simulink model "TST_DrvDem_SelectParameter"  (R2016b)
settings: Solver=FixedStepDiscrete  StartTime=0.0  StopTime=simTime  FixedStep=sampleTime  RelTol=1e-3
values from neighbouring files (symbols this model uses):
  testCase = 1    [initTST_DrvDem_SelectParameter_001.m]    (also in initTST_DrvDem_SelectParameter_002.m = 2; initTST_DrvDem_SelectParameter_003.m = 3)
libraries: simulink x82, UnitTest_Lib x78
(part 1 of 3)
settings Model: Creator=zhengjinyan  LastModifiedBy=zhengjinyan
settings DebuggingCC: SignalRangeChecking=error

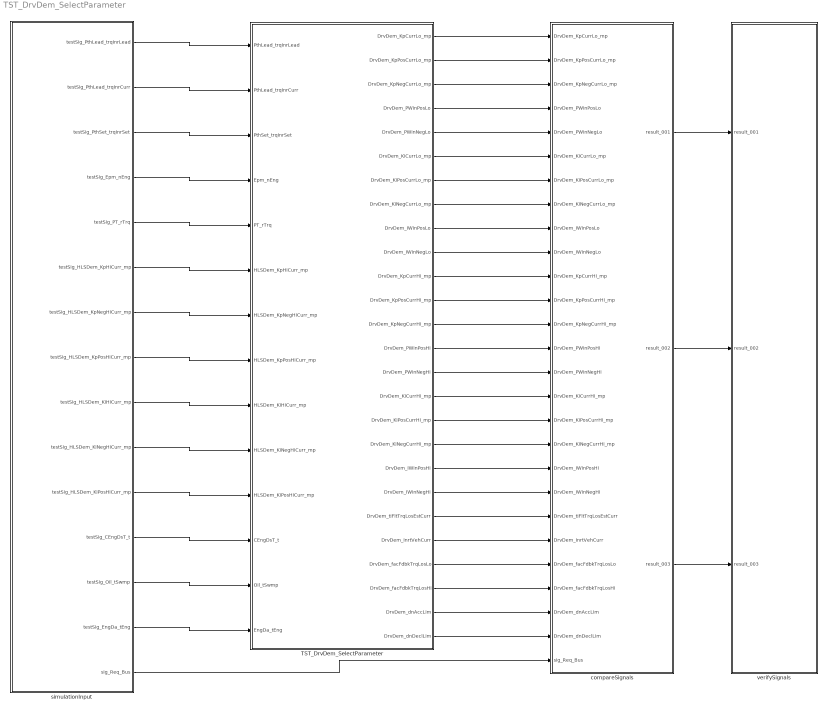
== system TST_DrvDem_SelectParameter ==
  TST_DrvDem_SelectParameter : Subsystem
  compareSignals : Subsystem
  simulationInput : Subsystem
  verifySignals : Subsystem
  wires:
  simulationInput/1(testSig_PthLead_trqInrLead) -> TST_DrvDem_SelectParameter/1(PthLead_trqInrLead)
  simulationInput/2(testSig_PthLead_trqInrCurr) -> TST_DrvDem_SelectParameter/2(PthLead_trqInrCurr)
  simulationInput/3(testSig_PthSet_trqInrSet) -> TST_DrvDem_SelectParameter/3(PthSet_trqInrSet)
  simulationInput/4(testSig_Epm_nEng) -> TST_DrvDem_SelectParameter/4(Epm_nEng)
  simulationInput/5(testSig_PT_rTrq) -> TST_DrvDem_SelectParameter/5(PT_rTrq)
  simulationInput/6(testSig_HLSDem_KpHiCurr_mp) -> TST_DrvDem_SelectParameter/6(HLSDem_KpHiCurr_mp)
  simulationInput/7(testSig_HLSDem_KpNegHiCurr_mp) -> TST_DrvDem_SelectParameter/7(HLSDem_KpNegHiCurr_mp)
  simulationInput/8(testSig_HLSDem_KpPosHiCurr_mp) -> TST_DrvDem_SelectParameter/8(HLSDem_KpPosHiCurr_mp)
  simulationInput/9(testSig_HLSDem_KiHiCurr_mp) -> TST_DrvDem_SelectParameter/9(HLSDem_KiHiCurr_mp)
  simulationInput/10(testSig_HLSDem_KiNegHiCurr_mp) -> TST_DrvDem_SelectParameter/10(HLSDem_KiNegHiCurr_mp)
  simulationInput/11(testSig_HLSDem_KiPosHiCurr_mp) -> TST_DrvDem_SelectParameter/11(HLSDem_KiPosHiCurr_mp)
  simulationInput/12(testSig_CEngDsT_t) -> TST_DrvDem_SelectParameter/12(CEngDsT_t)
  simulationInput/13(testSig_Oil_tSwmp) -> TST_DrvDem_SelectParameter/13(Oil_tSwmp)
  simulationInput/14(testSig_EngDa_tEng) -> TST_DrvDem_SelectParameter/14(EngDa_tEng)
  TST_DrvDem_SelectParameter/1(DrvDem_KpCurrLo_mp) -> compareSignals/1(DrvDem_KpCurrLo_mp)
  TST_DrvDem_SelectParameter/2(DrvDem_KpPosCurrLo_mp) -> compareSignals/2(DrvDem_KpPosCurrLo_mp)
  TST_DrvDem_SelectParameter/3(DrvDem_KpNegCurrLo_mp) -> compareSignals/3(DrvDem_KpNegCurrLo_mp)
  TST_DrvDem_SelectParameter/4(DrvDem_PWinPosLo) -> compareSignals/4(DrvDem_PWinPosLo)
  TST_DrvDem_SelectParameter/5(DrvDem_PWinNegLo) -> compareSignals/5(DrvDem_PWinNegLo)
  TST_DrvDem_SelectParameter/6(DrvDem_KiCurrLo_mp) -> compareSignals/6(DrvDem_KiCurrLo_mp)
  TST_DrvDem_SelectParameter/7(DrvDem_KiPosCurrLo_mp) -> compareSignals/7(DrvDem_KiPosCurrLo_mp)
  TST_DrvDem_SelectParameter/8(DrvDem_KiNegCurrLo_mp) -> compareSignals/8(DrvDem_KiNegCurrLo_mp)
  TST_DrvDem_SelectParameter/9(DrvDem_IWinPosLo) -> compareSignals/9(DrvDem_IWinPosLo)
  TST_DrvDem_SelectParameter/10(DrvDem_IWinNegLo) -> compareSignals/10(DrvDem_IWinNegLo)
  TST_DrvDem_SelectParameter/11(DrvDem_KpCurrHi_mp) -> compareSignals/11(DrvDem_KpCurrHi_mp)
  TST_DrvDem_SelectParameter/12(DrvDem_KpPosCurrHi_mp) -> compareSignals/12(DrvDem_KpPosCurrHi_mp)
  TST_DrvDem_SelectParameter/13(DrvDem_KpNegCurrHi_mp) -> compareSignals/13(DrvDem_KpNegCurrHi_mp)
  TST_DrvDem_SelectParameter/14(DrvDem_PWinPosHi) -> compareSignals/14(DrvDem_PWinPosHi)
  TST_DrvDem_SelectParameter/15(DrvDem_PWinNegHi) -> compareSignals/15(DrvDem_PWinNegHi)
  TST_DrvDem_SelectParameter/16(DrvDem_KiCurrHi_mp) -> compareSignals/16(DrvDem_KiCurrHi_mp)
  TST_DrvDem_SelectParameter/17(DrvDem_KiPosCurrHi_mp) -> compareSignals/17(DrvDem_KiPosCurrHi_mp)
  TST_DrvDem_SelectParameter/18(DrvDem_KiNegCurrHi_mp) -> compareSignals/18(DrvDem_KiNegCurrHi_mp)
  TST_DrvDem_SelectParameter/19(DrvDem_IWinPosHi) -> compareSignals/19(DrvDem_IWinPosHi)
  TST_DrvDem_SelectParameter/20(DrvDem_IWinNegHi) -> compareSignals/20(DrvDem_IWinNegHi)
  TST_DrvDem_SelectParameter/21(DrvDem_tiFltTrqLosEstCurr) -> compareSignals/21(DrvDem_tiFltTrqLosEstCurr)
  TST_DrvDem_SelectParameter/22(DrvDem_InrtVehCurr) -> compareSignals/22(DrvDem_InrtVehCurr)
  TST_DrvDem_SelectParameter/23(DrvDem_facFdbkTrqLosLo) -> compareSignals/23(DrvDem_facFdbkTrqLosLo)
  TST_DrvDem_SelectParameter/24(DrvDem_facFdbkTrqLosHi) -> compareSignals/24(DrvDem_facFdbkTrqLosHi)
  TST_DrvDem_SelectParameter/25(DrvDem_dnAccLim) -> compareSignals/25(DrvDem_dnAccLim)
  TST_DrvDem_SelectParameter/26(DrvDem_dnDeclLim) -> compareSignals/26(DrvDem_dnDeclLim)
  simulationInput/15(sig_Req_Bus) -> compareSignals/27(sig_Req_Bus)
  compareSignals/1(result_001) -> verifySignals/1(result_001)
  compareSignals/2(result_002) -> verifySignals/2(result_002)
  compareSignals/3(result_003) -> verifySignals/3(result_003)

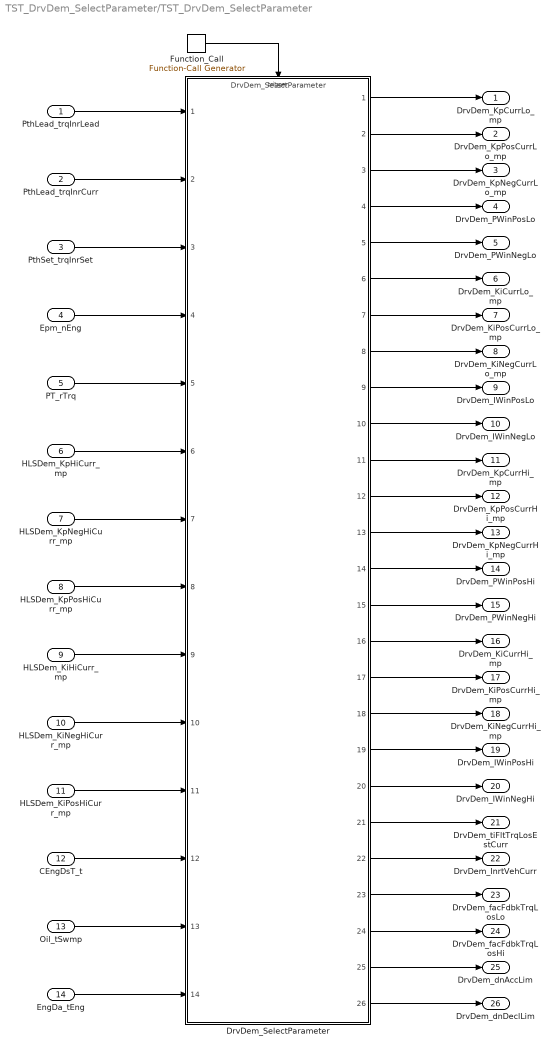
== system TST_DrvDem_SelectParameter/TST_DrvDem_SelectParameter ==
  PthLead_trqInrLead : Inport
  PthLead_trqInrCurr : Inport  Port=2
  PthSet_trqInrSet : Inport  Port=3
  Epm_nEng : Inport  Port=4
  PT_rTrq : Inport  Port=5
  HLSDem_KpHiCurr_mp : Inport  Port=6
  HLSDem_KpNegHiCurr_mp : Inport  Port=7
  HLSDem_KpPosHiCurr_mp : Inport  Port=8
  HLSDem_KiHiCurr_mp : Inport  Port=9
  HLSDem_KiNegHiCurr_mp : Inport  Port=10
  HLSDem_KiPosHiCurr_mp : Inport  Port=11
  CEngDsT_t : Inport  Port=12
  Oil_tSwmp : Inport  Port=13
  EngDa_tEng : Inport  Port=14
  DrvDem_SelectParameter : ModelReference  ModelNameDialog=DrvDem_SelectParameter  SimulationMode=Normal  ModelReferenceVersion=1.41  TriggerPortName=function  TriggerPortTriggerType=function-call  TriggerPortStatesWhenEnabling=held
  Function_Call : simulink/Ports & Subsystems/Function-Call Generator  sample_time=sampleTime  numberOfIterations=1
  DrvDem_KpCurrLo_mp : Outport
  DrvDem_KpPosCurrLo_mp : Outport  Port=2
  DrvDem_KpNegCurrLo_mp : Outport  Port=3
  DrvDem_PWinPosLo : Outport  Port=4
  DrvDem_PWinNegLo : Outport  Port=5
  DrvDem_KiCurrLo_mp : Outport  Port=6
  DrvDem_KiPosCurrLo_mp : Outport  Port=7
  DrvDem_KiNegCurrLo_mp : Outport  Port=8
  DrvDem_IWinPosLo : Outport  Port=9
  DrvDem_IWinNegLo : Outport  Port=10
  DrvDem_KpCurrHi_mp : Outport  Port=11
  DrvDem_KpPosCurrHi_mp : Outport  Port=12
  DrvDem_KpNegCurrHi_mp : Outport  Port=13
  DrvDem_PWinPosHi : Outport  Port=14
  DrvDem_PWinNegHi : Outport  Port=15
  DrvDem_KiCurrHi_mp : Outport  Port=16
  DrvDem_KiPosCurrHi_mp : Outport  Port=17
  DrvDem_KiNegCurrHi_mp : Outport  Port=18
  DrvDem_IWinPosHi : Outport  Port=19
  DrvDem_IWinNegHi : Outport  Port=20
  DrvDem_tiFltTrqLosEstCurr : Outport  Port=21
  DrvDem_InrtVehCurr : Outport  Port=22
  DrvDem_facFdbkTrqLosLo : Outport  Port=23
  DrvDem_facFdbkTrqLosHi : Outport  Port=24
  DrvDem_dnAccLim : Outport  Port=25
  DrvDem_dnDeclLim : Outport  Port=26
  wires:
  Function_Call/1 -> DrvDem_SelectParameter/Trigger
  PthLead_trqInrLead/1 -> DrvDem_SelectParameter/1
  PthLead_trqInrCurr/1 -> DrvDem_SelectParameter/2
  PthSet_trqInrSet/1 -> DrvDem_SelectParameter/3
  Epm_nEng/1 -> DrvDem_SelectParameter/4
  PT_rTrq/1 -> DrvDem_SelectParameter/5
  HLSDem_KpHiCurr_mp/1 -> DrvDem_SelectParameter/6
  HLSDem_KpNegHiCurr_mp/1 -> DrvDem_SelectParameter/7
  HLSDem_KpPosHiCurr_mp/1 -> DrvDem_SelectParameter/8
  HLSDem_KiHiCurr_mp/1 -> DrvDem_SelectParameter/9
  HLSDem_KiNegHiCurr_mp/1 -> DrvDem_SelectParameter/10
  HLSDem_KiPosHiCurr_mp/1 -> DrvDem_SelectParameter/11
  CEngDsT_t/1 -> DrvDem_SelectParameter/12
  Oil_tSwmp/1 -> DrvDem_SelectParameter/13
  EngDa_tEng/1 -> DrvDem_SelectParameter/14
  DrvDem_SelectParameter/1 -> DrvDem_KpCurrLo_mp/1
  DrvDem_SelectParameter/2 -> DrvDem_KpPosCurrLo_mp/1
  DrvDem_SelectParameter/3 -> DrvDem_KpNegCurrLo_mp/1
  DrvDem_SelectParameter/4 -> DrvDem_PWinPosLo/1
  DrvDem_SelectParameter/5 -> DrvDem_PWinNegLo/1
  DrvDem_SelectParameter/6 -> DrvDem_KiCurrLo_mp/1
  DrvDem_SelectParameter/7 -> DrvDem_KiPosCurrLo_mp/1
  DrvDem_SelectParameter/8 -> DrvDem_KiNegCurrLo_mp/1
  DrvDem_SelectParameter/9 -> DrvDem_IWinPosLo/1
  DrvDem_SelectParameter/10 -> DrvDem_IWinNegLo/1
  DrvDem_SelectParameter/11 -> DrvDem_KpCurrHi_mp/1
  DrvDem_SelectParameter/12 -> DrvDem_KpPosCurrHi_mp/1
  DrvDem_SelectParameter/13 -> DrvDem_KpNegCurrHi_mp/1
  DrvDem_SelectParameter/14 -> DrvDem_PWinPosHi/1
  DrvDem_SelectParameter/15 -> DrvDem_PWinNegHi/1
  DrvDem_SelectParameter/16 -> DrvDem_KiCurrHi_mp/1
  DrvDem_SelectParameter/17 -> DrvDem_KiPosCurrHi_mp/1
  DrvDem_SelectParameter/18 -> DrvDem_KiNegCurrHi_mp/1
  DrvDem_SelectParameter/19 -> DrvDem_IWinPosHi/1
  DrvDem_SelectParameter/20 -> DrvDem_IWinNegHi/1
  DrvDem_SelectParameter/21 -> DrvDem_tiFltTrqLosEstCurr/1
  DrvDem_SelectParameter/22 -> DrvDem_InrtVehCurr/1
  DrvDem_SelectParameter/23 -> DrvDem_facFdbkTrqLosLo/1
  DrvDem_SelectParameter/24 -> DrvDem_facFdbkTrqLosHi/1
  DrvDem_SelectParameter/25 -> DrvDem_dnAccLim/1
  DrvDem_SelectParameter/26 -> DrvDem_dnDeclLim/1

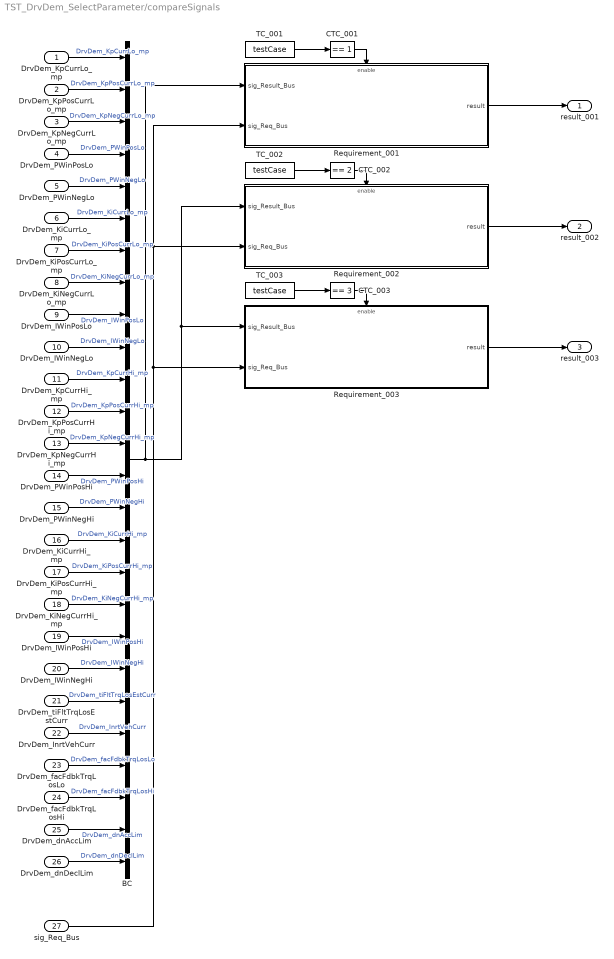
== system TST_DrvDem_SelectParameter/compareSignals ==
  DrvDem_KpCurrLo_mp : Inport
  DrvDem_KpPosCurrLo_mp : Inport  Port=2
  DrvDem_KpNegCurrLo_mp : Inport  Port=3
  DrvDem_PWinPosLo : Inport  Port=4
  DrvDem_PWinNegLo : Inport  Port=5
  DrvDem_KiCurrLo_mp : Inport  Port=6
  DrvDem_KiPosCurrLo_mp : Inport  Port=7
  DrvDem_KiNegCurrLo_mp : Inport  Port=8
  DrvDem_IWinPosLo : Inport  Port=9
  DrvDem_IWinNegLo : Inport  Port=10
  DrvDem_KpCurrHi_mp : Inport  Port=11
  DrvDem_KpPosCurrHi_mp : Inport  Port=12
  DrvDem_KpNegCurrHi_mp : Inport  Port=13
  DrvDem_PWinPosHi : Inport  Port=14
  DrvDem_PWinNegHi : Inport  Port=15
  DrvDem_KiCurrHi_mp : Inport  Port=16
  DrvDem_KiPosCurrHi_mp : Inport  Port=17
  DrvDem_KiNegCurrHi_mp : Inport  Port=18
  DrvDem_IWinPosHi : Inport  Port=19
  DrvDem_IWinNegHi : Inport  Port=20
  DrvDem_tiFltTrqLosEstCurr : Inport  Port=21
  DrvDem_InrtVehCurr : Inport  Port=22
  DrvDem_facFdbkTrqLosLo : Inport  Port=23
  DrvDem_facFdbkTrqLosHi : Inport  Port=24
  DrvDem_dnAccLim : Inport  Port=25
  DrvDem_dnDeclLim : Inport  Port=26
  sig_Req_Bus : Inport  Port=27
  BC : BusCreator  Inputs=26
  CTC_001 : simulink/Logic and Bit Operations/Compare To Constant  relop===  const=1  OutDataTypeStr=boolean
  CTC_002 : simulink/Logic and Bit Operations/Compare To Constant  relop===  const=2  OutDataTypeStr=boolean
  CTC_003 : simulink/Logic and Bit Operations/Compare To Constant  relop===  const=3  OutDataTypeStr=boolean
  Requirement_001 : Subsystem
  Requirement_002 : Subsystem
  Requirement_003 : Subsystem
  TC_001 : Constant  Value=testCase
  TC_002 : Constant  Value=testCase
  TC_003 : Constant  Value=testCase
  result_001 : Outport
  result_002 : Outport  Port=2
  result_003 : Outport  Port=3
  wires:
  DrvDem_KpCurrLo_mp/1 -> BC/1  "DrvDem_KpCurrLo_mp"
  DrvDem_KpPosCurrLo_mp/1 -> BC/2  "DrvDem_KpPosCurrLo_mp"
  DrvDem_KpNegCurrLo_mp/1 -> BC/3  "DrvDem_KpNegCurrLo_mp"
  DrvDem_PWinPosLo/1 -> BC/4  "DrvDem_PWinPosLo"
  DrvDem_PWinNegLo/1 -> BC/5  "DrvDem_PWinNegLo"
  DrvDem_KiCurrLo_mp/1 -> BC/6  "DrvDem_KiCurrLo_mp"
  DrvDem_KiPosCurrLo_mp/1 -> BC/7  "DrvDem_KiPosCurrLo_mp"
  DrvDem_KiNegCurrLo_mp/1 -> BC/8  "DrvDem_KiNegCurrLo_mp"
  DrvDem_IWinPosLo/1 -> BC/9  "DrvDem_IWinPosLo"
  DrvDem_IWinNegLo/1 -> BC/10  "DrvDem_IWinNegLo"
  DrvDem_KpCurrHi_mp/1 -> BC/11  "DrvDem_KpCurrHi_mp"
  DrvDem_KpPosCurrHi_mp/1 -> BC/12  "DrvDem_KpPosCurrHi_mp"
  DrvDem_KpNegCurrHi_mp/1 -> BC/13  "DrvDem_KpNegCurrHi_mp"
  DrvDem_PWinPosHi/1 -> BC/14  "DrvDem_PWinPosHi"
  DrvDem_PWinNegHi/1 -> BC/15  "DrvDem_PWinNegHi"
  DrvDem_KiCurrHi_mp/1 -> BC/16  "DrvDem_KiCurrHi_mp"
  DrvDem_KiPosCurrHi_mp/1 -> BC/17  "DrvDem_KiPosCurrHi_mp"
  DrvDem_KiNegCurrHi_mp/1 -> BC/18  "DrvDem_KiNegCurrHi_mp"
  DrvDem_IWinPosHi/1 -> BC/19  "DrvDem_IWinPosHi"
  DrvDem_IWinNegHi/1 -> BC/20  "DrvDem_IWinNegHi"
  DrvDem_tiFltTrqLosEstCurr/1 -> BC/21  "DrvDem_tiFltTrqLosEstCurr"
  DrvDem_InrtVehCurr/1 -> BC/22  "DrvDem_InrtVehCurr"
  DrvDem_facFdbkTrqLosLo/1 -> BC/23  "DrvDem_facFdbkTrqLosLo"
  DrvDem_facFdbkTrqLosHi/1 -> BC/24  "DrvDem_facFdbkTrqLosHi"
  DrvDem_dnAccLim/1 -> BC/25  "DrvDem_dnAccLim"
  DrvDem_dnDeclLim/1 -> BC/26  "DrvDem_dnDeclLim"
  TC_001/1 -> CTC_001/1
  CTC_001/1 -> Requirement_001/Enable
  sig_Req_Bus/1 -> Requirement_001/2(sig_Req_Bus), Requirement_002/2(sig_Req_Bus), Requirement_003/2(sig_Req_Bus)
  BC/1 -> Requirement_002/1(sig_Result_Bus), Requirement_003/1(sig_Result_Bus), Requirement_001/1(sig_Result_Bus)
  Requirement_001/1(result) -> result_001/1
  TC_002/1 -> CTC_002/1
  CTC_002/1 -> Requirement_002/Enable
  Requirement_002/1(result) -> result_002/1
  TC_003/1 -> CTC_003/1
  CTC_003/1 -> Requirement_003/Enable
  Requirement_003/1(result) -> result_003/1

== system TST_DrvDem_SelectParameter/simulationInput ==
  BS : BusSelector  OutputSignals=testSig_PthLead_trqInrLead,testSig_PthLead_trqInrCurr,testSig_PthSet_trqInrSet,testSig_Epm_nEng,testSig_PT_rTrq,testSig_HLSDem_KpHiCurr_mp,testSig_HLSDem_KpNegHiCurr_mp,testSig_HLSDem_KpPosHiCurr_mp,testSig_HLSDem_KiHiCurr_mp,testSig_HLSDem_KiNegHiCurr_mp,testSig_HLSDem_KiPosHiCurr_mp,testSig_CEngDsT_t,testSig_Oil_tSwmp,testSig_EngDa_tEng
  MPSw : MultiPortSwitch  SaturateOnIntegerOverflow=on  InputSameDT=on
  TestCase : Constant  Value=testCase
  testSignals_R001 : Subsystem
  testSignals_R002 : Subsystem
  testSignals_R003 : Subsystem
  testSig_PthLead_trqInrLead : Outport
  testSig_PthLead_trqInrCurr : Outport  Port=2
  testSig_PthSet_trqInrSet : Outport  Port=3
  testSig_Epm_nEng : Outport  Port=4
  testSig_PT_rTrq : Outport  Port=5
  testSig_HLSDem_KpHiCurr_mp : Outport  Port=6
  testSig_HLSDem_KpNegHiCurr_mp : Outport  Port=7
  testSig_HLSDem_KpPosHiCurr_mp : Outport  Port=8
  testSig_HLSDem_KiHiCurr_mp : Outport  Port=9
  testSig_HLSDem_KiNegHiCurr_mp : Outport  Port=10
  testSig_HLSDem_KiPosHiCurr_mp : Outport  Port=11
  testSig_CEngDsT_t : Outport  Port=12
  testSig_Oil_tSwmp : Outport  Port=13
  testSig_EngDa_tEng : Outport  Port=14
  sig_Req_Bus : Outport  Port=15
  wires:
  BS/1 -> testSig_PthLead_trqInrLead/1  "<testSig_PthLead_trqInrLead>"
  BS/2 -> testSig_PthLead_trqInrCurr/1  "<testSig_PthLead_trqInrCurr>"
  BS/3 -> testSig_PthSet_trqInrSet/1  "<testSig_PthSet_trqInrSet>"
  BS/4 -> testSig_Epm_nEng/1  "<testSig_Epm_nEng>"
  BS/5 -> testSig_PT_rTrq/1  "<testSig_PT_rTrq>"
  BS/6 -> testSig_HLSDem_KpHiCurr_mp/1  "<testSig_HLSDem_KpHiCurr_mp>"
  BS/7 -> testSig_HLSDem_KpNegHiCurr_mp/1  "<testSig_HLSDem_KpNegHiCurr_mp>"
  BS/8 -> testSig_HLSDem_KpPosHiCurr_mp/1  "<testSig_HLSDem_KpPosHiCurr_mp>"
  BS/9 -> testSig_HLSDem_KiHiCurr_mp/1  "<testSig_HLSDem_KiHiCurr_mp>"
  BS/10 -> testSig_HLSDem_KiNegHiCurr_mp/1  "<testSig_HLSDem_KiNegHiCurr_mp>"
  BS/11 -> testSig_HLSDem_KiPosHiCurr_mp/1  "<testSig_HLSDem_KiPosHiCurr_mp>"
  BS/12 -> testSig_CEngDsT_t/1  "<testSig_CEngDsT_t>"
  BS/13 -> testSig_Oil_tSwmp/1  "<testSig_Oil_tSwmp>"
  BS/14 -> testSig_EngDa_tEng/1  "<testSig_EngDa_tEng>"
  MPSw/1 -> BS/1, sig_Req_Bus/1
  TestCase/1 -> MPSw/1
  testSignals_R001/1(testSignals) -> MPSw/2
  testSignals_R002/1(testSignals) -> MPSw/3
  testSignals_R003/1(testSignals) -> MPSw/4

== system TST_DrvDem_SelectParameter/verifySignals ==
  result_001 : Inport
  result_002 : Inport  Port=2
  result_003 : Inport  Port=3
  Assertion_001 : Assertion  Enabled=off
  Assertion_002 : Assertion  Enabled=off
  Assertion_003 : Assertion  Enabled=off
  wires:
  result_001/1 -> Assertion_001/1
  result_002/1 -> Assertion_002/1
  result_003/1 -> Assertion_003/1

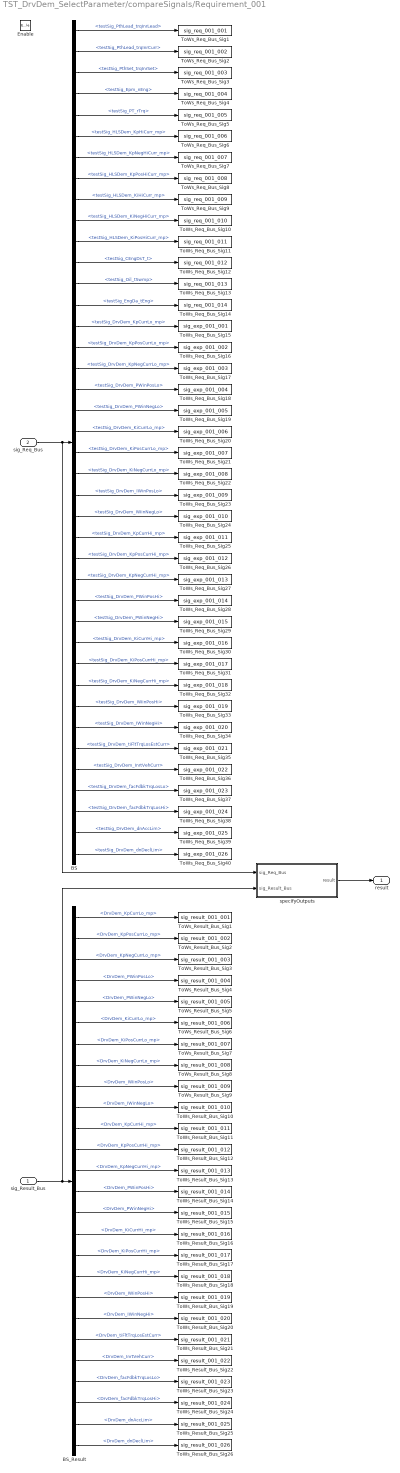
== system TST_DrvDem_SelectParameter/compareSignals/Requirement_001 ==
  sig_Result_Bus : Inport
  sig_Req_Bus : Inport  Port=2
  Enable : EnablePort
  BS : BusSelector  OutputSignals=testSig_PthLead_trqInrLead,testSig_PthLead_trqInrCurr,testSig_PthSet_trqInrSet,testSig_Epm_nEng,testSig_PT_rTrq,testSig_HLSDem_KpHiCurr_mp,testSig_HLSDem_KpNegHiCurr_mp,testSig_HLSDem_KpPosHiCurr_mp,testSig_HLSDem_KiHiCurr_mp,testSig_HLSDem_KiNegHiCurr_mp,testSig_HLSDem_KiPosHiCurr_mp,testSig_CEngDsT_t,testSig_Oil_tSwmp,testSig_EngDa_tEng,testSig_DrvDem_KpCurrLo_mp,testSig_DrvDem_KpPosCurrLo_mp,testSig_DrvDem_KpNegCurrLo_mp,testSig_DrvDem_PWinPosLo,testSig_DrvDem_PWinNegLo,testSig_DrvDem_KiCurrLo_mp,testSig_DrvDem_KiPosCurrLo_mp,testSig_DrvDem_KiNegCurrLo_mp,testSig_DrvDem_IWinPosLo,testSig_DrvDem_IWinNegLo,testSig_DrvDem_KpCurrHi_mp,testSig_DrvDem_KpPosCurrHi_mp,testSig_DrvDem_KpNegCurrHi_mp,testSig_DrvDem_PWinPosHi,testSig_DrvDem_PWinNegHi,testSig_DrvDem_KiCurrHi_mp,testSig_DrvDem_KiPosCurrHi_mp,testSig_DrvDem_KiNegCurrHi_mp,testSig_DrvDem_IWinPosHi,testSig_DrvDem_IWinNegHi,testSig_DrvDem_tiFltTrqLosEstCurr,testSig_DrvDem_InrtVehCurr,testSig_DrvDem_facFdbkTrqLosLo,testSig_DrvDem_facFdbkTrqLosHi,testSig_DrvDem_dnAccLim,testSig_DrvDem_dnDeclLim
  BS_Result : BusSelector  OutputSignals=DrvDem_KpCurrLo_mp,DrvDem_KpPosCurrLo_mp,DrvDem_KpNegCurrLo_mp,DrvDem_PWinPosLo,DrvDem_PWinNegLo,DrvDem_KiCurrLo_mp,DrvDem_KiPosCurrLo_mp,DrvDem_KiNegCurrLo_mp,DrvDem_IWinPosLo,DrvDem_IWinNegLo,DrvDem_KpCurrHi_mp,DrvDem_KpPosCurrHi_mp,DrvDem_KpNegCurrHi_mp,DrvDem_PWinPosHi,DrvDem_PWinNegHi,DrvDem_KiCurrHi_mp,DrvDem_KiPosCurrHi_mp,DrvDem_KiNegCurrHi_mp,DrvDem_IWinPosHi,DrvDem_IWinNegHi,DrvDem_tiFltTrqLosEstCurr,DrvDem_InrtVehCurr,DrvDem_facFdbkTrqLosLo,DrvDem_facFdbkTrqLosHi,DrvDem_dnAccLim,DrvDem_dnDeclLim
  ToWs_Req_Bus_Sig1 : ToWorkspace  VariableName=sig_req_001_001  SaveFormat=Structure With Time
  ToWs_Req_Bus_Sig10 : ToWorkspace  VariableName=sig_req_001_010  SaveFormat=Structure With Time
  ToWs_Req_Bus_Sig11 : ToWorkspace  VariableName=sig_req_001_011  SaveFormat=Structure With Time
  ToWs_Req_Bus_Sig12 : ToWorkspace  VariableName=sig_req_001_012  SaveFormat=Structure With Time
  ToWs_Req_Bus_Sig13 : ToWorkspace  VariableName=sig_req_001_013  SaveFormat=Structure With Time
  ToWs_Req_Bus_Sig14 : ToWorkspace  VariableName=sig_req_001_014  SaveFormat=Structure With Time
  ToWs_Req_Bus_Sig15 : ToWorkspace  VariableName=sig_exp_001_001  SaveFormat=Structure With Time
  ToWs_Req_Bus_Sig16 : ToWorkspace  VariableName=sig_exp_001_002  SaveFormat=Structure With Time
  ToWs_Req_Bus_Sig17 : ToWorkspace  VariableName=sig_exp_001_003  SaveFormat=Structure With Time
  ToWs_Req_Bus_Sig18 : ToWorkspace  VariableName=sig_exp_001_004  SaveFormat=Structure With Time
  ToWs_Req_Bus_Sig19 : ToWorkspace  VariableName=sig_exp_001_005  SaveFormat=Structure With Time
  ToWs_Req_Bus_Sig2 : ToWorkspace  VariableName=sig_req_001_002  SaveFormat=Structure With Time
  ToWs_Req_Bus_Sig20 : ToWorkspace  VariableName=sig_exp_001_006  SaveFormat=Structure With Time
  ToWs_Req_Bus_Sig21 : ToWorkspace  VariableName=sig_exp_001_007  SaveFormat=Structure With Time
  ToWs_Req_Bus_Sig22 : ToWorkspace  VariableName=sig_exp_001_008  SaveFormat=Structure With Time
  ToWs_Req_Bus_Sig23 : ToWorkspace  VariableName=sig_exp_001_009  SaveFormat=Structure With Time
  ToWs_Req_Bus_Sig24 : ToWorkspace  VariableName=sig_exp_001_010  SaveFormat=Structure With Time
  ToWs_Req_Bus_Sig25 : ToWorkspace  VariableName=sig_exp_001_011  SaveFormat=Structure With Time
  ToWs_Req_Bus_Sig26 : ToWorkspace  VariableName=sig_exp_001_012  SaveFormat=Structure With Time
  ToWs_Req_Bus_Sig27 : ToWorkspace  VariableName=sig_exp_001_013  SaveFormat=Structure With Time
  ToWs_Req_Bus_Sig28 : ToWorkspace  VariableName=sig_exp_001_014  SaveFormat=Structure With Time
  ToWs_Req_Bus_Sig29 : ToWorkspace  VariableName=sig_exp_001_015  SaveFormat=Structure With Time
  ToWs_Req_Bus_Sig3 : ToWorkspace  VariableName=sig_req_001_003  SaveFormat=Structure With Time
  ToWs_Req_Bus_Sig30 : ToWorkspace  VariableName=sig_exp_001_016  SaveFormat=Structure With Time
  ToWs_Req_Bus_Sig31 : ToWorkspace  VariableName=sig_exp_001_017  SaveFormat=Structure With Time
  ToWs_Req_Bus_Sig32 : ToWorkspace  VariableName=sig_exp_001_018  SaveFormat=Structure With Time
  ToWs_Req_Bus_Sig33 : ToWorkspace  VariableName=sig_exp_001_019  SaveFormat=Structure With Time
  ToWs_Req_Bus_Sig34 : ToWorkspace  VariableName=sig_exp_001_020  SaveFormat=Structure With Time
  ToWs_Req_Bus_Sig35 : ToWorkspace  VariableName=sig_exp_001_021  SaveFormat=Structure With Time
  ToWs_Req_Bus_Sig36 : ToWorkspace  VariableName=sig_exp_001_022  SaveFormat=Structure With Time
  ToWs_Req_Bus_Sig37 : ToWorkspace  VariableName=sig_exp_001_023  SaveFormat=Structure With Time
  ToWs_Req_Bus_Sig38 : ToWorkspace  VariableName=sig_exp_001_024  SaveFormat=Structure With Time
  ToWs_Req_Bus_Sig39 : ToWorkspace  VariableName=sig_exp_001_025  SaveFormat=Structure With Time
  ToWs_Req_Bus_Sig4 : ToWorkspace  VariableName=sig_req_001_004  SaveFormat=Structure With Time
  ToWs_Req_Bus_Sig40 : ToWorkspace  VariableName=sig_exp_001_026  SaveFormat=Structure With Time
  ToWs_Req_Bus_Sig5 : ToWorkspace  VariableName=sig_req_001_005  SaveFormat=Structure With Time
  ToWs_Req_Bus_Sig6 : ToWorkspace  VariableName=sig_req_001_006  SaveFormat=Structure With Time
  ToWs_Req_Bus_Sig7 : ToWorkspace  VariableName=sig_req_001_007  SaveFormat=Structure With Time
  ToWs_Req_Bus_Sig8 : ToWorkspace  VariableName=sig_req_001_008  SaveFormat=Structure With Time
  ToWs_Req_Bus_Sig9 : ToWorkspace  VariableName=sig_req_001_009  SaveFormat=Structure With Time
  ToWs_Result_Bus_Sig1 : ToWorkspace  VariableName=sig_result_001_001  SaveFormat=Structure With Time
  ToWs_Result_Bus_Sig10 : ToWorkspace  VariableName=sig_result_001_010  SaveFormat=Structure With Time
  ToWs_Result_Bus_Sig11 : ToWorkspace  VariableName=sig_result_001_011  SaveFormat=Structure With Time
  ToWs_Result_Bus_Sig12 : ToWorkspace  VariableName=sig_result_001_012  SaveFormat=Structure With Time
  ToWs_Result_Bus_Sig13 : ToWorkspace  VariableName=sig_result_001_013  SaveFormat=Structure With Time
  ToWs_Result_Bus_Sig14 : ToWorkspace  VariableName=sig_result_001_014  SaveFormat=Structure With Time
  ToWs_Result_Bus_Sig15 : ToWorkspace  VariableName=sig_result_001_015  SaveFormat=Structure With Time
  ToWs_Result_Bus_Sig16 : ToWorkspace  VariableName=sig_result_001_016  SaveFormat=Structure With Time
  ToWs_Result_Bus_Sig17 : ToWorkspace  VariableName=sig_result_001_017  SaveFormat=Structure With Time
  ToWs_Result_Bus_Sig18 : ToWorkspace  VariableName=sig_result_001_018  SaveFormat=Structure With Time
  ToWs_Result_Bus_Sig19 : ToWorkspace  VariableName=sig_result_001_019  SaveFormat=Structure With Time
  ToWs_Result_Bus_Sig2 : ToWorkspace  VariableName=sig_result_001_002  SaveFormat=Structure With Time
  ToWs_Result_Bus_Sig20 : ToWorkspace  VariableName=sig_result_001_020  SaveFormat=Structure With Time
  ToWs_Result_Bus_Sig21 : ToWorkspace  VariableName=sig_result_001_021  SaveFormat=Structure With Time
  ToWs_Result_Bus_Sig22 : ToWorkspace  VariableName=sig_result_001_022  SaveFormat=Structure With Time
  ToWs_Result_Bus_Sig23 : ToWorkspace  VariableName=sig_result_001_023  SaveFormat=Structure With Time
  ToWs_Result_Bus_Sig24 : ToWorkspace  VariableName=sig_result_001_024  SaveFormat=Structure With Time
  ToWs_Result_Bus_Sig25 : ToWorkspace  VariableName=sig_result_001_025  SaveFormat=Structure With Time
  ToWs_Result_Bus_Sig26 : ToWorkspace  VariableName=sig_result_001_026  SaveFormat=Structure With Time
  ToWs_Result_Bus_Sig3 : ToWorkspace  VariableName=sig_result_001_003  SaveFormat=Structure With Time
  ToWs_Result_Bus_Sig4 : ToWorkspace  VariableName=sig_result_001_004  SaveFormat=Structure With Time
  ToWs_Result_Bus_Sig5 : ToWorkspace  VariableName=sig_result_001_005  SaveFormat=Structure With Time
  ToWs_Result_Bus_Sig6 : ToWorkspace  VariableName=sig_result_001_006  SaveFormat=Structure With Time
  ToWs_Result_Bus_Sig7 : ToWorkspace  VariableName=sig_result_001_007  SaveFormat=Structure With Time
  ToWs_Result_Bus_Sig8 : ToWorkspace  VariableName=sig_result_001_008  SaveFormat=Structure With Time
  ToWs_Result_Bus_Sig9 : ToWorkspace  VariableName=sig_result_001_009  SaveFormat=Structure With Time
  specifyOutputs : Subsystem
  result : Outport
  wires:
  sig_Req_Bus/1 -> BS/1, specifyOutputs/1(sig_Req_Bus)
  BS/1 -> ToWs_Req_Bus_Sig1/1  "<testSig_PthLead_trqInrLead>"
  BS/2 -> ToWs_Req_Bus_Sig2/1  "<testSig_PthLead_trqInrCurr>"
  BS/3 -> ToWs_Req_Bus_Sig3/1  "<testSig_PthSet_trqInrSet>"
  BS/4 -> ToWs_Req_Bus_Sig4/1  "<testSig_Epm_nEng>"
  BS/5 -> ToWs_Req_Bus_Sig5/1  "<testSig_PT_rTrq>"
  BS/6 -> ToWs_Req_Bus_Sig6/1  "<testSig_HLSDem_KpHiCurr_mp>"
  BS/7 -> ToWs_Req_Bus_Sig7/1  "<testSig_HLSDem_KpNegHiCurr_mp>"
  BS/8 -> ToWs_Req_Bus_Sig8/1  "<testSig_HLSDem_KpPosHiCurr_mp>"
  BS/9 -> ToWs_Req_Bus_Sig9/1  "<testSig_HLSDem_KiHiCurr_mp>"
  BS/10 -> ToWs_Req_Bus_Sig10/1  "<testSig_HLSDem_KiNegHiCurr_mp>"
  BS/11 -> ToWs_Req_Bus_Sig11/1  "<testSig_HLSDem_KiPosHiCurr_mp>"
  BS/12 -> ToWs_Req_Bus_Sig12/1  "<testSig_CEngDsT_t>"
  BS/13 -> ToWs_Req_Bus_Sig13/1  "<testSig_Oil_tSwmp>"
  BS/14 -> ToWs_Req_Bus_Sig14/1  "<testSig_EngDa_tEng>"
  BS/15 -> ToWs_Req_Bus_Sig15/1  "<testSig_DrvDem_KpCurrLo_mp>"
  BS/16 -> ToWs_Req_Bus_Sig16/1  "<testSig_DrvDem_KpPosCurrLo_mp>"
  BS/17 -> ToWs_Req_Bus_Sig17/1  "<testSig_DrvDem_KpNegCurrLo_mp>"
  BS/18 -> ToWs_Req_Bus_Sig18/1  "<testSig_DrvDem_PWinPosLo>"
  BS/19 -> ToWs_Req_Bus_Sig19/1  "<testSig_DrvDem_PWinNegLo>"
  BS/20 -> ToWs_Req_Bus_Sig20/1  "<testSig_DrvDem_KiCurrLo_mp>"
  BS/21 -> ToWs_Req_Bus_Sig21/1  "<testSig_DrvDem_KiPosCurrLo_mp>"
  BS/22 -> ToWs_Req_Bus_Sig22/1  "<testSig_DrvDem_KiNegCurrLo_mp>"
  BS/23 -> ToWs_Req_Bus_Sig23/1  "<testSig_DrvDem_IWinPosLo>"
  BS/24 -> ToWs_Req_Bus_Sig24/1  "<testSig_DrvDem_IWinNegLo>"
  BS/25 -> ToWs_Req_Bus_Sig25/1  "<testSig_DrvDem_KpCurrHi_mp>"
  BS/26 -> ToWs_Req_Bus_Sig26/1  "<testSig_DrvDem_KpPosCurrHi_mp>"
  BS/27 -> ToWs_Req_Bus_Sig27/1  "<testSig_DrvDem_KpNegCurrHi_mp>"
  BS/28 -> ToWs_Req_Bus_Sig28/1  "<testSig_DrvDem_PWinPosHi>"
  BS/29 -> ToWs_Req_Bus_Sig29/1  "<testSig_DrvDem_PWinNegHi>"
  BS/30 -> ToWs_Req_Bus_Sig30/1  "<testSig_DrvDem_KiCurrHi_mp>"
  BS/31 -> ToWs_Req_Bus_Sig31/1  "<testSig_DrvDem_KiPosCurrHi_mp>"
  BS/32 -> ToWs_Req_Bus_Sig32/1  "<testSig_DrvDem_KiNegCurrHi_mp>"
  BS/33 -> ToWs_Req_Bus_Sig33/1  "<testSig_DrvDem_IWinPosHi>"
  BS/34 -> ToWs_Req_Bus_Sig34/1  "<testSig_DrvDem_IWinNegHi>"
  BS/35 -> ToWs_Req_Bus_Sig35/1  "<testSig_DrvDem_tiFltTrqLosEstCurr>"
  BS/36 -> ToWs_Req_Bus_Sig36/1  "<testSig_DrvDem_InrtVehCurr>"
  BS/37 -> ToWs_Req_Bus_Sig37/1  "<testSig_DrvDem_facFdbkTrqLosLo>"
  BS/38 -> ToWs_Req_Bus_Sig38/1  "<testSig_DrvDem_facFdbkTrqLosHi>"
  BS/39 -> ToWs_Req_Bus_Sig39/1  "<testSig_DrvDem_dnAccLim>"
  BS/40 -> ToWs_Req_Bus_Sig40/1  "<testSig_DrvDem_dnDeclLim>"
  sig_Result_Bus/1 -> BS_Result/1, specifyOutputs/2(sig_Result_Bus)
  BS_Result/1 -> ToWs_Result_Bus_Sig1/1  "<DrvDem_KpCurrLo_mp>"
  BS_Result/2 -> ToWs_Result_Bus_Sig2/1  "<DrvDem_KpPosCurrLo_mp>"
  BS_Result/3 -> ToWs_Result_Bus_Sig3/1  "<DrvDem_KpNegCurrLo_mp>"
  BS_Result/4 -> ToWs_Result_Bus_Sig4/1  "<DrvDem_PWinPosLo>"
  BS_Result/5 -> ToWs_Result_Bus_Sig5/1  "<DrvDem_PWinNegLo>"
  BS_Result/6 -> ToWs_Result_Bus_Sig6/1  "<DrvDem_KiCurrLo_mp>"
  BS_Result/7 -> ToWs_Result_Bus_Sig7/1  "<DrvDem_KiPosCurrLo_mp>"
  BS_Result/8 -> ToWs_Result_Bus_Sig8/1  "<DrvDem_KiNegCurrLo_mp>"
  BS_Result/9 -> ToWs_Result_Bus_Sig9/1  "<DrvDem_IWinPosLo>"
  BS_Result/10 -> ToWs_Result_Bus_Sig10/1  "<DrvDem_IWinNegLo>"
  BS_Result/11 -> ToWs_Result_Bus_Sig11/1  "<DrvDem_KpCurrHi_mp>"
  BS_Result/12 -> ToWs_Result_Bus_Sig12/1  "<DrvDem_KpPosCurrHi_mp>"
  BS_Result/13 -> ToWs_Result_Bus_Sig13/1  "<DrvDem_KpNegCurrHi_mp>"
  BS_Result/14 -> ToWs_Result_Bus_Sig14/1  "<DrvDem_PWinPosHi>"
  BS_Result/15 -> ToWs_Result_Bus_Sig15/1  "<DrvDem_PWinNegHi>"
  BS_Result/16 -> ToWs_Result_Bus_Sig16/1  "<DrvDem_KiCurrHi_mp>"
  BS_Result/17 -> ToWs_Result_Bus_Sig17/1  "<DrvDem_KiPosCurrHi_mp>"
  BS_Result/18 -> ToWs_Result_Bus_Sig18/1  "<DrvDem_KiNegCurrHi_mp>"
  BS_Result/19 -> ToWs_Result_Bus_Sig19/1  "<DrvDem_IWinPosHi>"
  BS_Result/20 -> ToWs_Result_Bus_Sig20/1  "<DrvDem_IWinNegHi>"
  BS_Result/21 -> ToWs_Result_Bus_Sig21/1  "<DrvDem_tiFltTrqLosEstCurr>"
  BS_Result/22 -> ToWs_Result_Bus_Sig22/1  "<DrvDem_InrtVehCurr>"
  BS_Result/23 -> ToWs_Result_Bus_Sig23/1  "<DrvDem_facFdbkTrqLosLo>"
  BS_Result/24 -> ToWs_Result_Bus_Sig24/1  "<DrvDem_facFdbkTrqLosHi>"
  BS_Result/25 -> ToWs_Result_Bus_Sig25/1  "<DrvDem_dnAccLim>"
  BS_Result/26 -> ToWs_Result_Bus_Sig26/1  "<DrvDem_dnDeclLim>"
  specifyOutputs/1(result) -> result/1

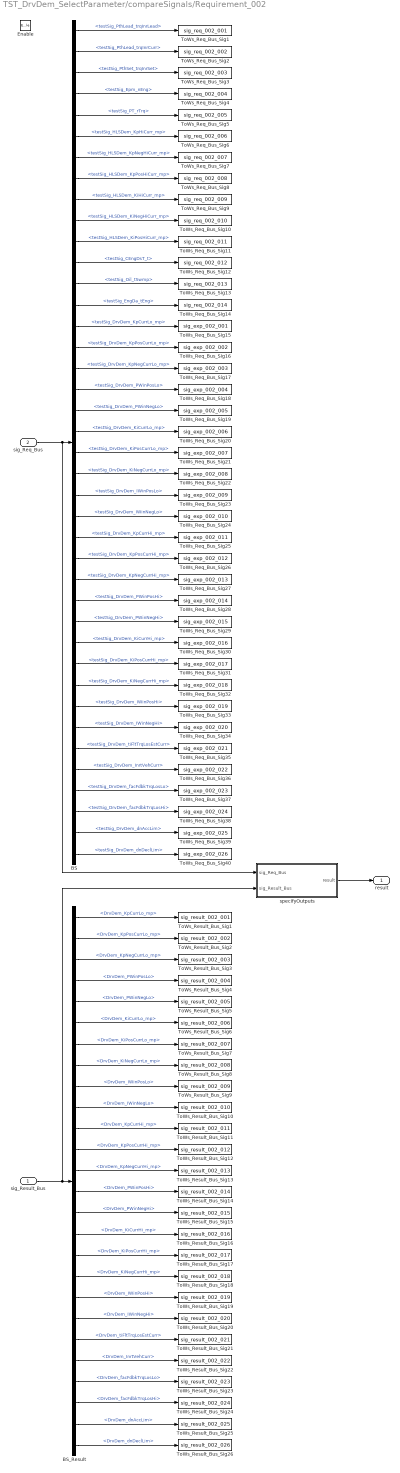
== system TST_DrvDem_SelectParameter/compareSignals/Requirement_002 ==
  sig_Result_Bus : Inport
  sig_Req_Bus : Inport  Port=2
  Enable : EnablePort
  BS : BusSelector  OutputSignals=testSig_PthLead_trqInrLead,testSig_PthLead_trqInrCurr,testSig_PthSet_trqInrSet,testSig_Epm_nEng,testSig_PT_rTrq,testSig_HLSDem_KpHiCurr_mp,testSig_HLSDem_KpNegHiCurr_mp,testSig_HLSDem_KpPosHiCurr_mp,testSig_HLSDem_KiHiCurr_mp,testSig_HLSDem_KiNegHiCurr_mp,testSig_HLSDem_KiPosHiCurr_mp,testSig_CEngDsT_t,testSig_Oil_tSwmp,testSig_EngDa_tEng,testSig_DrvDem_KpCurrLo_mp,testSig_DrvDem_KpPosCurrLo_mp,testSig_DrvDem_KpNegCurrLo_mp,testSig_DrvDem_PWinPosLo,testSig_DrvDem_PWinNegLo,testSig_DrvDem_KiCurrLo_mp,testSig_DrvDem_KiPosCurrLo_mp,testSig_DrvDem_KiNegCurrLo_mp,testSig_DrvDem_IWinPosLo,testSig_DrvDem_IWinNegLo,testSig_DrvDem_KpCurrHi_mp,testSig_DrvDem_KpPosCurrHi_mp,testSig_DrvDem_KpNegCurrHi_mp,testSig_DrvDem_PWinPosHi,testSig_DrvDem_PWinNegHi,testSig_DrvDem_KiCurrHi_mp,testSig_DrvDem_KiPosCurrHi_mp,testSig_DrvDem_KiNegCurrHi_mp,testSig_DrvDem_IWinPosHi,testSig_DrvDem_IWinNegHi,testSig_DrvDem_tiFltTrqLosEstCurr,testSig_DrvDem_InrtVehCurr,testSig_DrvDem_facFdbkTrqLosLo,testSig_DrvDem_facFdbkTrqLosHi,testSig_DrvDem_dnAccLim,testSig_DrvDem_dnDeclLim
  BS_Result : BusSelector  OutputSignals=DrvDem_KpCurrLo_mp,DrvDem_KpPosCurrLo_mp,DrvDem_KpNegCurrLo_mp,DrvDem_PWinPosLo,DrvDem_PWinNegLo,DrvDem_KiCurrLo_mp,DrvDem_KiPosCurrLo_mp,DrvDem_KiNegCurrLo_mp,DrvDem_IWinPosLo,DrvDem_IWinNegLo,DrvDem_KpCurrHi_mp,DrvDem_KpPosCurrHi_mp,DrvDem_KpNegCurrHi_mp,DrvDem_PWinPosHi,DrvDem_PWinNegHi,DrvDem_KiCurrHi_mp,DrvDem_KiPosCurrHi_mp,DrvDem_KiNegCurrHi_mp,DrvDem_IWinPosHi,DrvDem_IWinNegHi,DrvDem_tiFltTrqLosEstCurr,DrvDem_InrtVehCurr,DrvDem_facFdbkTrqLosLo,DrvDem_facFdbkTrqLosHi,DrvDem_dnAccLim,DrvDem_dnDeclLim
  ToWs_Req_Bus_Sig1 : ToWorkspace  VariableName=sig_req_002_001  SaveFormat=Structure With Time
  ToWs_Req_Bus_Sig10 : ToWorkspace  VariableName=sig_req_002_010  SaveFormat=Structure With Time
  ToWs_Req_Bus_Sig11 : ToWorkspace  VariableName=sig_req_002_011  SaveFormat=Structure With Time
  ToWs_Req_Bus_Sig12 : ToWorkspace  VariableName=sig_req_002_012  SaveFormat=Structure With Time
  ToWs_Req_Bus_Sig13 : ToWorkspace  VariableName=sig_req_002_013  SaveFormat=Structure With Time
  ToWs_Req_Bus_Sig14 : ToWorkspace  VariableName=sig_req_002_014  SaveFormat=Structure With Time
  ToWs_Req_Bus_Sig15 : ToWorkspace  VariableName=sig_exp_002_001  SaveFormat=Structure With Time
  ToWs_Req_Bus_Sig16 : ToWorkspace  VariableName=sig_exp_002_002  SaveFormat=Structure With Time
  ToWs_Req_Bus_Sig17 : ToWorkspace  VariableName=sig_exp_002_003  SaveFormat=Structure With Time
  ToWs_Req_Bus_Sig18 : ToWorkspace  VariableName=sig_exp_002_004  SaveFormat=Structure With Time
  ToWs_Req_Bus_Sig19 : ToWorkspace  VariableName=sig_exp_002_005  SaveFormat=Structure With Time
  ToWs_Req_Bus_Sig2 : ToWorkspace  VariableName=sig_req_002_002  SaveFormat=Structure With Time
  ToWs_Req_Bus_Sig20 : ToWorkspace  VariableName=sig_exp_002_006  SaveFormat=Structure With Time
  ToWs_Req_Bus_Sig21 : ToWorkspace  VariableName=sig_exp_002_007  SaveFormat=Structure With Time
  ToWs_Req_Bus_Sig22 : ToWorkspace  VariableName=sig_exp_002_008  SaveFormat=Structure With Time
  ToWs_Req_Bus_Sig23 : ToWorkspace  VariableName=sig_exp_002_009  SaveFormat=Structure With Time
  ToWs_Req_Bus_Sig24 : ToWorkspace  VariableName=sig_exp_002_010  SaveFormat=Structure With Time
  ToWs_Req_Bus_Sig25 : ToWorkspace  VariableName=sig_exp_002_011  SaveFormat=Structure With Time
  ToWs_Req_Bus_Sig26 : ToWorkspace  VariableName=sig_exp_002_012  SaveFormat=Structure With Time
  ToWs_Req_Bus_Sig27 : ToWorkspace  VariableName=sig_exp_002_013  SaveFormat=Structure With Time
  ToWs_Req_Bus_Sig28 : ToWorkspace  VariableName=sig_exp_002_014  SaveFormat=Structure With Time
  ToWs_Req_Bus_Sig29 : ToWorkspace  VariableName=sig_exp_002_015  SaveFormat=Structure With Time
  ToWs_Req_Bus_Sig3 : ToWorkspace  VariableName=sig_req_002_003  SaveFormat=Structure With Time
  ToWs_Req_Bus_Sig30 : ToWorkspace  VariableName=sig_exp_002_016  SaveFormat=Structure With Time
  ToWs_Req_Bus_Sig31 : ToWorkspace  VariableName=sig_exp_002_017  SaveFormat=Structure With Time
  ToWs_Req_Bus_Sig32 : ToWorkspace  VariableName=sig_exp_002_018  SaveFormat=Structure With Time
  ToWs_Req_Bus_Sig33 : ToWorkspace  VariableName=sig_exp_002_019  SaveFormat=Structure With Time
  ToWs_Req_Bus_Sig34 : ToWorkspace  VariableName=sig_exp_002_020  SaveFormat=Structure With Time
  ToWs_Req_Bus_Sig35 : ToWorkspace  VariableName=sig_exp_002_021  SaveFormat=Structure With Time
  ToWs_Req_Bus_Sig36 : ToWorkspace  VariableName=sig_exp_002_022  SaveFormat=Structure With Time
  ToWs_Req_Bus_Sig37 : ToWorkspace  VariableName=sig_exp_002_023  SaveFormat=Structure With Time
  ToWs_Req_Bus_Sig38 : ToWorkspace  VariableName=sig_exp_002_024  SaveFormat=Structure With Time
  ToWs_Req_Bus_Sig39 : ToWorkspace  VariableName=sig_exp_002_025  SaveFormat=Structure With Time
  ToWs_Req_Bus_Sig4 : ToWorkspace  VariableName=sig_req_002_004  SaveFormat=Structure With Time
  ToWs_Req_Bus_Sig40 : ToWorkspace  VariableName=sig_exp_002_026  SaveFormat=Structure With Time
  ToWs_Req_Bus_Sig5 : ToWorkspace  VariableName=sig_req_002_005  SaveFormat=Structure With Time
  ToWs_Req_Bus_Sig6 : ToWorkspace  VariableName=sig_req_002_006  SaveFormat=Structure With Time
  ToWs_Req_Bus_Sig7 : ToWorkspace  VariableName=sig_req_002_007  SaveFormat=Structure With Time
  ToWs_Req_Bus_Sig8 : ToWorkspace  VariableName=sig_req_002_008  SaveFormat=Structure With Time
  ToWs_Req_Bus_Sig9 : ToWorkspace  VariableName=sig_req_002_009  SaveFormat=Structure With Time
  ToWs_Result_Bus_Sig1 : ToWorkspace  VariableName=sig_result_002_001  SaveFormat=Structure With Time
  ToWs_Result_Bus_Sig10 : ToWorkspace  VariableName=sig_result_002_010  SaveFormat=Structure With Time
  ToWs_Result_Bus_Sig11 : ToWorkspace  VariableName=sig_result_002_011  SaveFormat=Structure With Time
  ToWs_Result_Bus_Sig12 : ToWorkspace  VariableName=sig_result_002_012  SaveFormat=Structure With Time
  ToWs_Result_Bus_Sig13 : ToWorkspace  VariableName=sig_result_002_013  SaveFormat=Structure With Time
  ToWs_Result_Bus_Sig14 : ToWorkspace  VariableName=sig_result_002_014  SaveFormat=Structure With Time
  ToWs_Result_Bus_Sig15 : ToWorkspace  VariableName=sig_result_002_015  SaveFormat=Structure With Time
  ToWs_Result_Bus_Sig16 : ToWorkspace  VariableName=sig_result_002_016  SaveFormat=Structure With Time
  ToWs_Result_Bus_Sig17 : ToWorkspace  VariableName=sig_result_002_017  SaveFormat=Structure With Time
  ToWs_Result_Bus_Sig18 : ToWorkspace  VariableName=sig_result_002_018  SaveFormat=Structure With Time
  ToWs_Result_Bus_Sig19 : ToWorkspace  VariableName=sig_result_002_019  SaveFormat=Structure With Time
  ToWs_Result_Bus_Sig2 : ToWorkspace  VariableName=sig_result_002_002  SaveFormat=Structure With Time
  ToWs_Result_Bus_Sig20 : ToWorkspace  VariableName=sig_result_002_020  SaveFormat=Structure With Time
  ToWs_Result_Bus_Sig21 : ToWorkspace  VariableName=sig_result_002_021  SaveFormat=Structure With Time
  ToWs_Result_Bus_Sig22 : ToWorkspace  VariableName=sig_result_002_022  SaveFormat=Structure With Time
  ToWs_Result_Bus_Sig23 : ToWorkspace  VariableName=sig_result_002_023  SaveFormat=Structure With Time
  ToWs_Result_Bus_Sig24 : ToWorkspace  VariableName=sig_result_002_024  SaveFormat=Structure With Time
  ToWs_Result_Bus_Sig25 : ToWorkspace  VariableName=sig_result_002_025  SaveFormat=Structure With Time
  ToWs_Result_Bus_Sig26 : ToWorkspace  VariableName=sig_result_002_026  SaveFormat=Structure With Time
  ToWs_Result_Bus_Sig3 : ToWorkspace  VariableName=sig_result_002_003  SaveFormat=Structure With Time
  ToWs_Result_Bus_Sig4 : ToWorkspace  VariableName=sig_result_002_004  SaveFormat=Structure With Time
  ToWs_Result_Bus_Sig5 : ToWorkspace  VariableName=sig_result_002_005  SaveFormat=Structure With Time
  ToWs_Result_Bus_Sig6 : ToWorkspace  VariableName=sig_result_002_006  SaveFormat=Structure With Time
  ToWs_Result_Bus_Sig7 : ToWorkspace  VariableName=sig_result_002_007  SaveFormat=Structure With Time
  ToWs_Result_Bus_Sig8 : ToWorkspace  VariableName=sig_result_002_008  SaveFormat=Structure With Time
  ToWs_Result_Bus_Sig9 : ToWorkspace  VariableName=sig_result_002_009  SaveFormat=Structure With Time
  specifyOutputs : Subsystem
  result : Outport
  wires:
  sig_Req_Bus/1 -> BS/1, specifyOutputs/1(sig_Req_Bus)
  BS/1 -> ToWs_Req_Bus_Sig1/1  "<testSig_PthLead_trqInrLead>"
  BS/2 -> ToWs_Req_Bus_Sig2/1  "<testSig_PthLead_trqInrCurr>"
  BS/3 -> ToWs_Req_Bus_Sig3/1  "<testSig_PthSet_trqInrSet>"
  BS/4 -> ToWs_Req_Bus_Sig4/1  "<testSig_Epm_nEng>"
  BS/5 -> ToWs_Req_Bus_Sig5/1  "<testSig_PT_rTrq>"
  BS/6 -> ToWs_Req_Bus_Sig6/1  "<testSig_HLSDem_KpHiCurr_mp>"
  BS/7 -> ToWs_Req_Bus_Sig7/1  "<testSig_HLSDem_KpNegHiCurr_mp>"
  BS/8 -> ToWs_Req_Bus_Sig8/1  "<testSig_HLSDem_KpPosHiCurr_mp>"
  BS/9 -> ToWs_Req_Bus_Sig9/1  "<testSig_HLSDem_KiHiCurr_mp>"
  BS/10 -> ToWs_Req_Bus_Sig10/1  "<testSig_HLSDem_KiNegHiCurr_mp>"
  BS/11 -> ToWs_Req_Bus_Sig11/1  "<testSig_HLSDem_KiPosHiCurr_mp>"
  BS/12 -> ToWs_Req_Bus_Sig12/1  "<testSig_CEngDsT_t>"
  BS/13 -> ToWs_Req_Bus_Sig13/1  "<testSig_Oil_tSwmp>"
  BS/14 -> ToWs_Req_Bus_Sig14/1  "<testSig_EngDa_tEng>"
  BS/15 -> ToWs_Req_Bus_Sig15/1  "<testSig_DrvDem_KpCurrLo_mp>"
  BS/16 -> ToWs_Req_Bus_Sig16/1  "<testSig_DrvDem_KpPosCurrLo_mp>"
  BS/17 -> ToWs_Req_Bus_Sig17/1  "<testSig_DrvDem_KpNegCurrLo_mp>"
  BS/18 -> ToWs_Req_Bus_Sig18/1  "<testSig_DrvDem_PWinPosLo>"
  BS/19 -> ToWs_Req_Bus_Sig19/1  "<testSig_DrvDem_PWinNegLo>"
  BS/20 -> ToWs_Req_Bus_Sig20/1  "<testSig_DrvDem_KiCurrLo_mp>"
  BS/21 -> ToWs_Req_Bus_Sig21/1  "<testSig_DrvDem_KiPosCurrLo_mp>"
  BS/22 -> ToWs_Req_Bus_Sig22/1  "<testSig_DrvDem_KiNegCurrLo_mp>"
  BS/23 -> ToWs_Req_Bus_Sig23/1  "<testSig_DrvDem_IWinPosLo>"
  BS/24 -> ToWs_Req_Bus_Sig24/1  "<testSig_DrvDem_IWinNegLo>"
  BS/25 -> ToWs_Req_Bus_Sig25/1  "<testSig_DrvDem_KpCurrHi_mp>"
  BS/26 -> ToWs_Req_Bus_Sig26/1  "<testSig_DrvDem_KpPosCurrHi_mp>"
  BS/27 -> ToWs_Req_Bus_Sig27/1  "<testSig_DrvDem_KpNegCurrHi_mp>"
  BS/28 -> ToWs_Req_Bus_Sig28/1  "<testSig_DrvDem_PWinPosHi>"
  BS/29 -> ToWs_Req_Bus_Sig29/1  "<testSig_DrvDem_PWinNegHi>"
  BS/30 -> ToWs_Req_Bus_Sig30/1  "<testSig_DrvDem_KiCurrHi_mp>"
  BS/31 -> ToWs_Req_Bus_Sig31/1  "<testSig_DrvDem_KiPosCurrHi_mp>"
  BS/32 -> ToWs_Req_Bus_Sig32/1  "<testSig_DrvDem_KiNegCurrHi_mp>"
  BS/33 -> ToWs_Req_Bus_Sig33/1  "<testSig_DrvDem_IWinPosHi>"
  BS/34 -> ToWs_Req_Bus_Sig34/1  "<testSig_DrvDem_IWinNegHi>"
  BS/35 -> ToWs_Req_Bus_Sig35/1  "<testSig_DrvDem_tiFltTrqLosEstCurr>"
  BS/36 -> ToWs_Req_Bus_Sig36/1  "<testSig_DrvDem_InrtVehCurr>"
  BS/37 -> ToWs_Req_Bus_Sig37/1  "<testSig_DrvDem_facFdbkTrqLosLo>"
  BS/38 -> ToWs_Req_Bus_Sig38/1  "<testSig_DrvDem_facFdbkTrqLosHi>"
  BS/39 -> ToWs_Req_Bus_Sig39/1  "<testSig_DrvDem_dnAccLim>"
  BS/40 -> ToWs_Req_Bus_Sig40/1  "<testSig_DrvDem_dnDeclLim>"
  sig_Result_Bus/1 -> BS_Result/1, specifyOutputs/2(sig_Result_Bus)
  BS_Result/1 -> ToWs_Result_Bus_Sig1/1  "<DrvDem_KpCurrLo_mp>"
  BS_Result/2 -> ToWs_Result_Bus_Sig2/1  "<DrvDem_KpPosCurrLo_mp>"
  BS_Result/3 -> ToWs_Result_Bus_Sig3/1  "<DrvDem_KpNegCurrLo_mp>"
  BS_Result/4 -> ToWs_Result_Bus_Sig4/1  "<DrvDem_PWinPosLo>"
  BS_Result/5 -> ToWs_Result_Bus_Sig5/1  "<DrvDem_PWinNegLo>"
  BS_Result/6 -> ToWs_Result_Bus_Sig6/1  "<DrvDem_KiCurrLo_mp>"
  BS_Result/7 -> ToWs_Result_Bus_Sig7/1  "<DrvDem_KiPosCurrLo_mp>"
  BS_Result/8 -> ToWs_Result_Bus_Sig8/1  "<DrvDem_KiNegCurrLo_mp>"
  BS_Result/9 -> ToWs_Result_Bus_Sig9/1  "<DrvDem_IWinPosLo>"
  BS_Result/10 -> ToWs_Result_Bus_Sig10/1  "<DrvDem_IWinNegLo>"
  BS_Result/11 -> ToWs_Result_Bus_Sig11/1  "<DrvDem_KpCurrHi_mp>"
  BS_Result/12 -> ToWs_Result_Bus_Sig12/1  "<DrvDem_KpPosCurrHi_mp>"
  BS_Result/13 -> ToWs_Result_Bus_Sig13/1  "<DrvDem_KpNegCurrHi_mp>"
  BS_Result/14 -> ToWs_Result_Bus_Sig14/1  "<DrvDem_PWinPosHi>"
  BS_Result/15 -> ToWs_Result_Bus_Sig15/1  "<DrvDem_PWinNegHi>"
  BS_Result/16 -> ToWs_Result_Bus_Sig16/1  "<DrvDem_KiCurrHi_mp>"
  BS_Result/17 -> ToWs_Result_Bus_Sig17/1  "<DrvDem_KiPosCurrHi_mp>"
  BS_Result/18 -> ToWs_Result_Bus_Sig18/1  "<DrvDem_KiNegCurrHi_mp>"
  BS_Result/19 -> ToWs_Result_Bus_Sig19/1  "<DrvDem_IWinPosHi>"
  BS_Result/20 -> ToWs_Result_Bus_Sig20/1  "<DrvDem_IWinNegHi>"
  BS_Result/21 -> ToWs_Result_Bus_Sig21/1  "<DrvDem_tiFltTrqLosEstCurr>"
  BS_Result/22 -> ToWs_Result_Bus_Sig22/1  "<DrvDem_InrtVehCurr>"
  BS_Result/23 -> ToWs_Result_Bus_Sig23/1  "<DrvDem_facFdbkTrqLosLo>"
  BS_Result/24 -> ToWs_Result_Bus_Sig24/1  "<DrvDem_facFdbkTrqLosHi>"
  BS_Result/25 -> ToWs_Result_Bus_Sig25/1  "<DrvDem_dnAccLim>"
  BS_Result/26 -> ToWs_Result_Bus_Sig26/1  "<DrvDem_dnDeclLim>"
  specifyOutputs/1(result) -> result/1
